simulink model "DARM"  (Simulink 7.5)
settings: Solver=ode45  StartTime=0.0  StopTime=10.0  RelTol=1e-3
values from neighbouring files (symbols this model uses):
  ifoParams = evalin('base', 'ifoParams')    [darmNbParams.m]
libraries: cstblocks x132, NbLibrary x29
(part 1 of 2)
settings Model: Creator=kissel  LastModifiedBy=controls
settings CodeAppCC: CustomSymbolStrType=$N$R$M_T

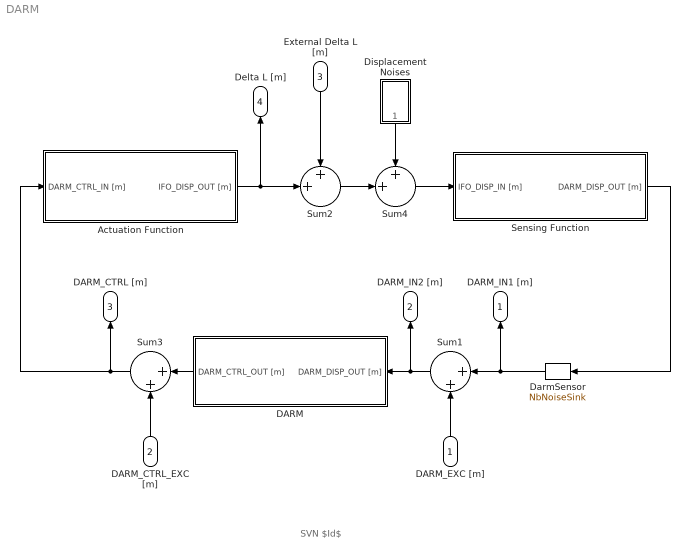
== system DARM ==
  note: SVN $Id$
  DARM_EXC [m] : Inport
  DARM_CTRL_EXC [m] : Inport  Port=2
  External Delta L [m] : Inport  Port=3
  Actuation Function : Subsystem
  DARM : Subsystem
  DarmSensor : NbLibrary/NbNoiseSink  Tag=NbNoiseSink  SystemSampleTime=-1  dof='DARM'
      settings: AttributesFormatString=%<Tag>
  Displacement Noises : Subsystem
  Sensing Function : Subsystem
  Sum1 : Sum  Inputs=|++
  Sum2 : Sum  Inputs=++|
  Sum3 : Sum  Inputs=|++
  Sum4 : Sum  Inputs=++|
  DARM_IN1 [m] : Outport
  DARM_IN2 [m] : Outport  Port=2
  DARM_CTRL [m] : Outport  Port=3
  Delta L [m] : Outport  Port=4
  wires:
  Sum1/1 -> DARM/1(DARM_DISP_OUT [m]), DARM_IN2 [m]/1
  Sensing Function/1(DARM_DISP_OUT [m]) -> DarmSensor/1
  DARM_EXC [m]/1 -> Sum1/2
  Actuation Function/1(IFO_DISP_OUT [m]) -> Sum2/2, Delta L [m]/1
  External Delta L [m]/1 -> Sum2/1
  Sum3/1 -> Actuation Function/1(DARM_CTRL_IN [m]), DARM_CTRL [m]/1
  DARM_CTRL_EXC [m]/1 -> Sum3/2
  DARM/1(DARM_CTRL_OUT [m]) -> Sum3/1
  DarmSensor/1 -> Sum1/1, DARM_IN1 [m]/1
  Sum2/1 -> Sum4/2
  Sum4/1 -> Sensing Function/1(IFO_DISP_IN [m])
  Displacement Noises/1(Out [m]) -> Sum4/1

== system DARM/Actuation Function ==
  DARM_CTRL_IN [m] : Inport
  ETMX : Subsystem
  ETMY : Subsystem
  IFO2OPTIC : Subsystem
  Subtract : Sum  Inputs=+-
  IFO_DISP_OUT [m] : Outport
  wires:
  IFO2OPTIC/1(ETMX_CTRL_OUT [m]) -> ETMX/1(ETMX_CTRL_IN [m])
  IFO2OPTIC/2(ETMY_CTRL_OUT [m]) -> ETMY/1(ETMY_CTRL_IN [m])
  ETMX/1(ETM_Displacement [m]) -> Subtract/1
  ETMY/1(ETM_Displacement [m]) -> Subtract/2
  DARM_CTRL_IN [m]/1 -> IFO2OPTIC/1(DARM_CTRL_IN [m])
  Subtract/1 -> IFO_DISP_OUT [m]/1

== system DARM/DARM ==
  DARM_DISP_OUT [m] : Inport
  FM1 : cstblocks/LTI System  Description=FlexTf: ifoParams.dig.darm(1).frd  SystemSampleTime=-1  sys=ifoParams.dig.darm(1).ss  IC=[]
      settings: AttributesFormatString=%<Description>
  FM10 : cstblocks/LTI System  SystemSampleTime=-1  sys=ifoParams.dig.darm(10).ss  IC=[]
  FM2 : cstblocks/LTI System  Description=FlexTf: ifoParams.dig.darm(2).frd  SystemSampleTime=-1  sys=ifoParams.dig.darm(2).ss  IC=[]
      settings: AttributesFormatString=%<Description>
  FM3 : cstblocks/LTI System  SystemSampleTime=-1  sys=ifoParams.dig.darm(3).ss  IC=[]
  FM4 : cstblocks/LTI System  SystemSampleTime=-1  sys=ifoParams.dig.darm(4).ss  IC=[]
  FM5 : cstblocks/LTI System  SystemSampleTime=-1  sys=ifoParams.dig.darm(5).ss  IC=[]
  FM6 : cstblocks/LTI System  SystemSampleTime=-1  sys=ifoParams.dig.darm(6).ss  IC=[]
  FM7 : cstblocks/LTI System  SystemSampleTime=-1  sys=ifoParams.dig.darm(7).ss  IC=[]
  FM8 : cstblocks/LTI System  SystemSampleTime=-1  sys=ifoParams.dig.darm(8).ss  IC=[]
  FM9 : cstblocks/LTI System  SystemSampleTime=-1  sys=ifoParams.dig.darm(9).ss  IC=[]
  Gain2 : Gain  Gain=ifoParams.dig.darmGain
  DARM_CTRL_OUT [m] : Outport
  wires:
  FM1/1 -> FM2/1
  FM2/1 -> FM3/1
  FM3/1 -> FM4/1
  FM4/1 -> FM5/1
  FM6/1 -> FM7/1
  FM7/1 -> FM8/1
  FM8/1 -> FM9/1
  FM9/1 -> FM10/1
  DARM_DISP_OUT [m]/1 -> FM1/1
  FM10/1 -> Gain2/1
  Gain2/1 -> DARM_CTRL_OUT [m]/1
  FM5/1 -> FM6/1

== system DARM/Displacement Noises ==
  DarmMeters : NbLibrary/NbNoiseCal  Tag=NbNoiseCal  SystemSampleTime=-1  dof='DARM'  unit='displacement [m/rtHz]'
      settings: AttributesFormatString=%<Tag>
  ScatteredLightRing : NbLibrary/NbNoiseSource  Tag=NbNoiseSource  SystemSampleTime=-1  group='Scattered Light Ring'  asd=ifoParams.darmNb.scatteredLightRing
      settings: AttributesFormatString=%<Tag>
  Sum2 : Sum
  Out [m] : Outport
  wires:
  DarmMeters/1 -> Sum2/1
  Sum2/1 -> Out [m]/1
  ScatteredLightRing/1 -> Sum2/2

== system DARM/Sensing Function ==
  IFO_DISP_IN [m] : Inport
  ADC : Subsystem
  DCPD Analog Electronics : Subsystem
  DCPD Signal Conditioning : Subsystem
  IFO2PD : Subsystem
  LaserAm : NbLibrary/NbNoiseSource  Tag=NbNoiseSource  SystemSampleTime=-1  group='Laser Intensity'  asd=ifoParams.darmNb.laserAm
      settings: AttributesFormatString=%<Tag>
  LaserPm : NbLibrary/NbNoiseSource  Tag=NbNoiseSource  SystemSampleTime=-1  group='Laser Frequency'  asd=ifoParams.darmNb.laserPm
      settings: AttributesFormatString=%<Tag>
  Mich : NbLibrary/NbNoiseSource  Tag=NbNoiseSource  SystemSampleTime=-1  group='MICH Coupling'  asd=ifoParams.darmNb.mich
      settings: AttributesFormatString=%<Tag>
  OscAm : NbLibrary/NbNoiseSource  Tag=NbNoiseSource  SystemSampleTime=-1  group='Oscillator Amplitude'  asd=ifoParams.darmNb.oscAm
      settings: AttributesFormatString=%<Tag>
  OscPm : NbLibrary/NbNoiseSource  Tag=NbNoiseSource  SystemSampleTime=-1  group='Oscillator Phase'  asd=ifoParams.darmNb.oscPm
      settings: AttributesFormatString=%<Tag>
  PD2IFO : Subsystem
  Quantum : NbLibrary/NbNoiseSource  Tag=NbNoiseSource  SystemSampleTime=-1  group='Quantum'  asd=ifoParams.darmNb.quantum
      settings: AttributesFormatString=%<Tag>
  Sum2 : Sum  Inputs=+++++++
  ifoResponse : cstblocks/LTI System  Description=FlexTf: ifoParams.sens.ifoResponse.frd  SystemSampleTime=-1  sys=ifoParams.sens.ifoResponse.ss  IC=[]
      settings: AttributesFormatString=%<Description>
  DARM_DISP_OUT [m] : Outport
  wires:
  IFO2PD/1(PD1_OUT [W]) -> DCPD Analog Electronics/1(PD1_IN [W])
  IFO2PD/2(PD2_OUT [W]) -> DCPD Analog Electronics/2(PD2_IN [W])
  IFO_DISP_IN [m]/1 -> ifoResponse/1
  DCPD Signal Conditioning/1(PD1_OUT [m]) -> PD2IFO/1(PD1_IN1 [m])
  DCPD Signal Conditioning/2(PD2_OUT [m]) -> PD2IFO/2(PD2_IN [m])
  PD2IFO/1(DARM_DISP_OUT [m]) -> DARM_DISP_OUT [m]/1
  DCPD Analog Electronics/1(PD1_OUT [V]) -> ADC/1(PD1_IN1 [V])
  DCPD Analog Electronics/2(PD2_OUT [V]) -> ADC/2(PD2_IN [V])
  ADC/1(PD1_OUT [ct]) -> DCPD Signal Conditioning/1(PD1_IN [ct])
  ADC/2(PD2_OUT [ct]) -> DCPD Signal Conditioning/2(PD2_IN [ct])
  ifoResponse/1 -> Sum2/1
  Sum2/1 -> IFO2PD/1(IFO_OUT [W])
  LaserAm/1 -> Sum2/2
  LaserPm/1 -> Sum2/3
  OscAm/1 -> Sum2/4
  OscPm/1 -> Sum2/5
  Quantum/1 -> Sum2/6
  Mich/1 -> Sum2/7

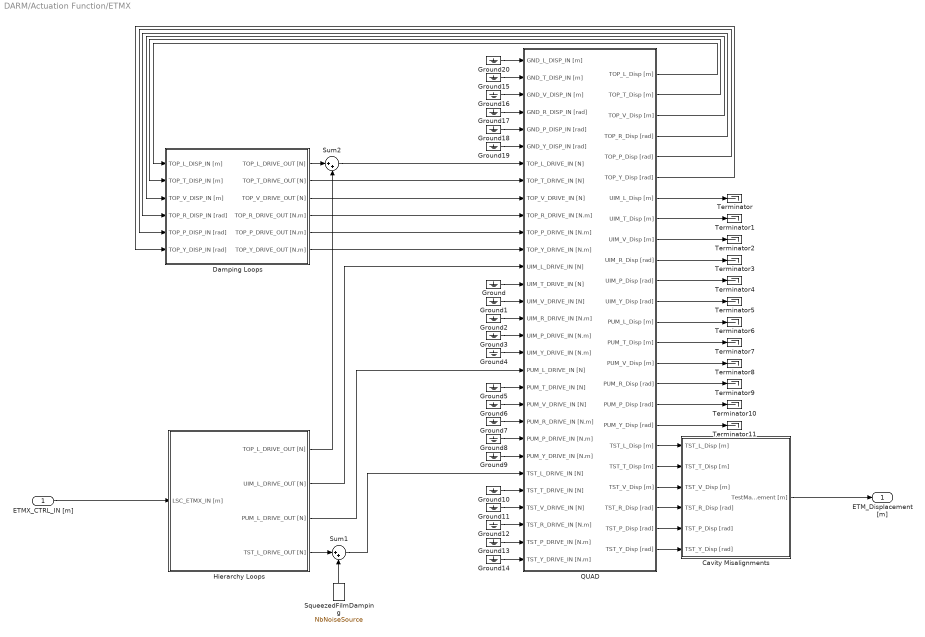
== system DARM/Actuation Function/ETMX ==
  ETMX_CTRL_IN [m] : Inport
  Cavity Misalignments : Subsystem
  Damping Loops : Subsystem
  Ground{,1..20} (21 alike) : Ground
  Hierarchy Loops : Subsystem
  QUAD : Subsystem
  SqueezedFilmDamping : NbLibrary/NbNoiseSource  Tag=NbNoiseSource  SystemSampleTime=-1  group='Squeezed Film Damping'  asd=ifoParams.darmNb.squeezedFilmDamping
      settings: AttributesFormatString=%<Tag>
  Sum1 : Sum  Inputs=|++
  Sum2 : Sum  Inputs=|++
  Terminator{,1..11} (12 alike) : Terminator
  ETM_Displacement [m] : Outport
  wires:
  QUAD/1(TOP_L_Disp [m]) -> Damping Loops/1(TOP_L_DISP_IN [m])
  QUAD/2(TOP_T_Disp [m]) -> Damping Loops/2(TOP_T_DISP_IN [m])
  QUAD/3(TOP_V_Disp [m]) -> Damping Loops/3(TOP_V_DISP_IN [m])
  QUAD/4(TOP_R_Disp [rad]) -> Damping Loops/4(TOP_R_DISP_IN [rad])
  QUAD/5(TOP_P_Disp [rad]) -> Damping Loops/5(TOP_P_DISP_IN [rad])
  QUAD/6(TOP_Y_Disp [rad]) -> Damping Loops/6(TOP_Y_DISP_IN [rad])
  QUAD/7(UIM_L_Disp [m]) -> Terminator/1
  QUAD/8(UIM_T_Disp [m]) -> Terminator1/1
  QUAD/9(UIM_V_Disp [m]) -> Terminator2/1
  QUAD/10(UIM_R_Disp [rad]) -> Terminator3/1
  QUAD/11(UIM_P_Disp [rad]) -> Terminator4/1
  QUAD/12(UIM_Y_Disp [rad]) -> Terminator5/1
  QUAD/13(PUM_L_Disp [m]) -> Terminator6/1
  QUAD/14(PUM_T_Disp [m]) -> Terminator7/1
  QUAD/15(PUM_V_Disp [m]) -> Terminator8/1
  QUAD/16(PUM_R_Disp [rad]) -> Terminator9/1
  QUAD/17(PUM_P_Disp [rad]) -> Terminator10/1
  QUAD/18(PUM_Y_Disp [rad]) -> Terminator11/1
  QUAD/19(TST_L_Disp [m]) -> Cavity Misalignments/1(TST_L_Disp [m])
  QUAD/20(TST_T_Disp [m]) -> Cavity Misalignments/2(TST_T_Disp [m])
  QUAD/21(TST_V_Disp [m]) -> Cavity Misalignments/3(TST_V_Disp [m])
  QUAD/22(TST_R_Disp [rad]) -> Cavity Misalignments/4(TST_R_Disp [rad])
  QUAD/23(TST_P_Disp [rad]) -> Cavity Misalignments/5(TST_P_Disp [rad])
  QUAD/24(TST_Y_Disp [rad]) -> Cavity Misalignments/6(TST_Y_Disp [rad])
  Ground/1 -> QUAD/14(UIM_T_DRIVE_IN [N])
  Ground1/1 -> QUAD/15(UIM_V_DRIVE_IN [N])
  Ground4/1 -> QUAD/18(UIM_Y_DRIVE_IN [N.m])
  Ground3/1 -> QUAD/17(UIM_P_DRIVE_IN [N.m])
  Ground2/1 -> QUAD/16(UIM_R_DRIVE_IN [N.m])
  Ground5/1 -> QUAD/20(PUM_T_DRIVE_IN [N])
  Ground6/1 -> QUAD/21(PUM_V_DRIVE_IN [N])
  Ground7/1 -> QUAD/22(PUM_R_DRIVE_IN [N.m])
  Ground8/1 -> QUAD/23(PUM_P_DRIVE_IN [N.m])
  Ground9/1 -> QUAD/24(PUM_Y_DRIVE_IN [N.m])
  Ground10/1 -> QUAD/26(TST_T_DRIVE_IN [N])
  Ground11/1 -> QUAD/27(TST_V_DRIVE_IN [N])
  Ground12/1 -> QUAD/28(TST_R_DRIVE_IN [N.m])
  Ground13/1 -> QUAD/29(TST_P_DRIVE_IN [N.m])
  Ground14/1 -> QUAD/30(TST_Y_DRIVE_IN [N.m])
  Cavity Misalignments/1(TestMass_L_Displacement [m]) -> ETM_Displacement [m]/1
  Hierarchy Loops/3(PUM_L_DRIVE_OUT [N]) -> QUAD/19(PUM_L_DRIVE_IN [N])
  Hierarchy Loops/2(UIM_L_DRIVE_OUT [N]) -> QUAD/13(UIM_L_DRIVE_IN [N])
  Damping Loops/2(TOP_T_DRIVE_OUT [N]) -> QUAD/8(TOP_T_DRIVE_IN [N])
  Damping Loops/3(TOP_V_DRIVE_OUT [N]) -> QUAD/9(TOP_V_DRIVE_IN [N])
  Damping Loops/4(TOP_R_DRIVE_OUT [N.m]) -> QUAD/10(TOP_R_DRIVE_IN [N.m])
  Damping Loops/5(TOP_P_DRIVE_OUT [N.m]) -> QUAD/11(TOP_P_DRIVE_IN [N.m])
  Damping Loops/6(TOP_Y_DRIVE_OUT [N.m]) -> QUAD/12(TOP_Y_DRIVE_IN [N.m])
  Damping Loops/1(TOP_L_DRIVE_OUT [N]) -> Sum2/1
  Hierarchy Loops/1(TOP_L_DRIVE_OUT [N]) -> Sum2/2
  Sum2/1 -> QUAD/7(TOP_L_DRIVE_IN [N])
  ETMX_CTRL_IN [m]/1 -> Hierarchy Loops/1(LSC_ETMX_IN [m])
  Ground20/1 -> QUAD/1(GND_L_DISP_IN [m])
  Ground15/1 -> QUAD/2(GND_T_DISP_IN [m])
  Ground16/1 -> QUAD/3(GND_V_DISP_IN [m])
  Ground17/1 -> QUAD/4(GND_R_DISP_IN [rad])
  Ground18/1 -> QUAD/5(GND_P_DISP_IN [rad])
  Ground19/1 -> QUAD/6(GND_Y_DISP_IN [rad])
  Sum1/1 -> QUAD/25(TST_L_DRIVE_IN [N])
  Hierarchy Loops/4(TST_L_DRIVE_OUT [N]) -> Sum1/1
  SqueezedFilmDamping/1 -> Sum1/2

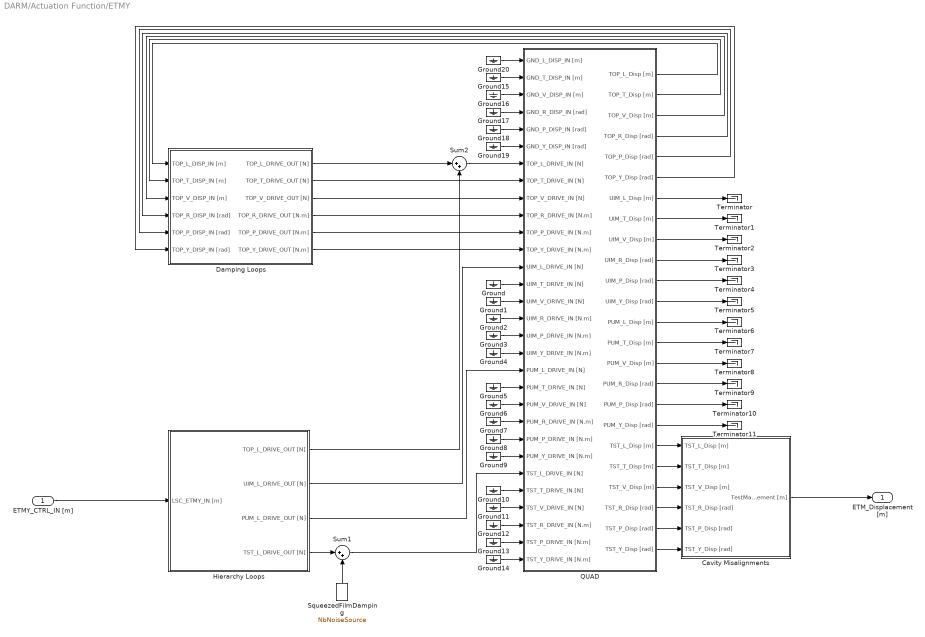
== system DARM/Actuation Function/ETMY ==
  ETMY_CTRL_IN [m] : Inport
  Cavity Misalignments : Subsystem
  Damping Loops : Subsystem
  Ground{,1..20} (21 alike) : Ground
  Hierarchy Loops : Subsystem
  QUAD : Subsystem
  SqueezedFilmDamping : NbLibrary/NbNoiseSource  Tag=NbNoiseSource  SystemSampleTime=-1  group='Squeezed Film Damping'  asd=ifoParams.darmNb.squeezedFilmDamping
      settings: AttributesFormatString=%<Tag>
  Sum1 : Sum  Inputs=|++
  Sum2 : Sum  Inputs=|++
  Terminator{,1..11} (12 alike) : Terminator
  ETM_Displacement [m] : Outport
  wires:
  QUAD/1(TOP_L_Disp [m]) -> Damping Loops/1(TOP_L_DISP_IN [m])
  QUAD/2(TOP_T_Disp [m]) -> Damping Loops/2(TOP_T_DISP_IN [m])
  QUAD/3(TOP_V_Disp [m]) -> Damping Loops/3(TOP_V_DISP_IN [m])
  QUAD/4(TOP_R_Disp [rad]) -> Damping Loops/4(TOP_R_DISP_IN [rad])
  QUAD/5(TOP_P_Disp [rad]) -> Damping Loops/5(TOP_P_DISP_IN [rad])
  QUAD/6(TOP_Y_Disp [rad]) -> Damping Loops/6(TOP_Y_DISP_IN [rad])
  QUAD/7(UIM_L_Disp [m]) -> Terminator/1
  QUAD/8(UIM_T_Disp [m]) -> Terminator1/1
  QUAD/9(UIM_V_Disp [m]) -> Terminator2/1
  QUAD/10(UIM_R_Disp [rad]) -> Terminator3/1
  QUAD/11(UIM_P_Disp [rad]) -> Terminator4/1
  QUAD/12(UIM_Y_Disp [rad]) -> Terminator5/1
  QUAD/13(PUM_L_Disp [m]) -> Terminator6/1
  QUAD/14(PUM_T_Disp [m]) -> Terminator7/1
  QUAD/15(PUM_V_Disp [m]) -> Terminator8/1
  QUAD/16(PUM_R_Disp [rad]) -> Terminator9/1
  QUAD/17(PUM_P_Disp [rad]) -> Terminator10/1
  QUAD/18(PUM_Y_Disp [rad]) -> Terminator11/1
  QUAD/19(TST_L_Disp [m]) -> Cavity Misalignments/1(TST_L_Disp [m])
  QUAD/20(TST_T_Disp [m]) -> Cavity Misalignments/2(TST_T_Disp [m])
  QUAD/21(TST_V_Disp [m]) -> Cavity Misalignments/3(TST_V_Disp [m])
  QUAD/22(TST_R_Disp [rad]) -> Cavity Misalignments/4(TST_R_Disp [rad])
  QUAD/23(TST_P_Disp [rad]) -> Cavity Misalignments/5(TST_P_Disp [rad])
  QUAD/24(TST_Y_Disp [rad]) -> Cavity Misalignments/6(TST_Y_Disp [rad])
  Ground/1 -> QUAD/14(UIM_T_DRIVE_IN [N])
  Ground1/1 -> QUAD/15(UIM_V_DRIVE_IN [N])
  Ground4/1 -> QUAD/18(UIM_Y_DRIVE_IN [N.m])
  Ground3/1 -> QUAD/17(UIM_P_DRIVE_IN [N.m])
  Ground2/1 -> QUAD/16(UIM_R_DRIVE_IN [N.m])
  Ground5/1 -> QUAD/20(PUM_T_DRIVE_IN [N])
  Ground6/1 -> QUAD/21(PUM_V_DRIVE_IN [N])
  Ground7/1 -> QUAD/22(PUM_R_DRIVE_IN [N.m])
  Ground8/1 -> QUAD/23(PUM_P_DRIVE_IN [N.m])
  Ground9/1 -> QUAD/24(PUM_Y_DRIVE_IN [N.m])
  Ground10/1 -> QUAD/26(TST_T_DRIVE_IN [N])
  Ground11/1 -> QUAD/27(TST_V_DRIVE_IN [N])
  Ground12/1 -> QUAD/28(TST_R_DRIVE_IN [N.m])
  Ground13/1 -> QUAD/29(TST_P_DRIVE_IN [N.m])
  Ground14/1 -> QUAD/30(TST_Y_DRIVE_IN [N.m])
  Cavity Misalignments/1(TestMass_L_Displacement [m]) -> ETM_Displacement [m]/1
  Hierarchy Loops/3(PUM_L_DRIVE_OUT [N]) -> QUAD/19(PUM_L_DRIVE_IN [N])
  Hierarchy Loops/2(UIM_L_DRIVE_OUT [N]) -> QUAD/13(UIM_L_DRIVE_IN [N])
  Damping Loops/2(TOP_T_DRIVE_OUT [N]) -> QUAD/8(TOP_T_DRIVE_IN [N])
  Damping Loops/3(TOP_V_DRIVE_OUT [N]) -> QUAD/9(TOP_V_DRIVE_IN [N])
  Damping Loops/4(TOP_R_DRIVE_OUT [N.m]) -> QUAD/10(TOP_R_DRIVE_IN [N.m])
  Damping Loops/5(TOP_P_DRIVE_OUT [N.m]) -> QUAD/11(TOP_P_DRIVE_IN [N.m])
  Damping Loops/6(TOP_Y_DRIVE_OUT [N.m]) -> QUAD/12(TOP_Y_DRIVE_IN [N.m])
  Damping Loops/1(TOP_L_DRIVE_OUT [N]) -> Sum2/1
  Hierarchy Loops/1(TOP_L_DRIVE_OUT [N]) -> Sum2/2
  Sum2/1 -> QUAD/7(TOP_L_DRIVE_IN [N])
  ETMY_CTRL_IN [m]/1 -> Hierarchy Loops/1(LSC_ETMY_IN [m])
  Ground20/1 -> QUAD/1(GND_L_DISP_IN [m])
  Ground15/1 -> QUAD/2(GND_T_DISP_IN [m])
  Ground16/1 -> QUAD/3(GND_V_DISP_IN [m])
  Ground17/1 -> QUAD/4(GND_R_DISP_IN [rad])
  Ground18/1 -> QUAD/5(GND_P_DISP_IN [rad])
  Ground19/1 -> QUAD/6(GND_Y_DISP_IN [rad])
  Hierarchy Loops/4(TST_L_DRIVE_OUT [N]) -> Sum1/1
  SqueezedFilmDamping/1 -> Sum1/2
  Sum1/1 -> QUAD/25(TST_L_DRIVE_IN [N])

== system DARM/Actuation Function/IFO2OPTIC ==
  DARM_CTRL_IN [m] : Inport
  Gain3 : Gain  Gain=ifoParams.act.darm2etmx
  Gain4 : Gain  Gain=ifoParams.act.darm2etmy
  ETMX_CTRL_OUT [m] : Outport
  ETMY_CTRL_OUT [m] : Outport  Port=2
  wires:
  DARM_CTRL_IN [m]/1 -> Gain3/1, Gain4/1
  Gain3/1 -> ETMX_CTRL_OUT [m]/1
  Gain4/1 -> ETMY_CTRL_OUT [m]/1

== system DARM/Sensing Function/ADC ==
  note: ifoParams.sens.adcGain
      | [ct/V]
  PD1_IN1 [V] : Inport
  PD2_IN [V] : Inport  Port=2
  AdcPd1 : NbLibrary/NbNoiseSource  Tag=NbNoiseSource  SystemSampleTime=-1  group='ADC'  asd=ifoParams.darmNb.adc
      settings: AttributesFormatString=%<Tag>
  AdcPd2 : NbLibrary/NbNoiseSource  Tag=NbNoiseSource  SystemSampleTime=-1  group='ADC'  asd=ifoParams.darmNb.adc
      settings: AttributesFormatString=%<Tag>
  Gain1 : Gain  Gain=ifoParams.sens.adcGain
  Gain3 : Gain  Gain=ifoParams.sens.adcGain
  Sum2 : Sum  Inputs=++|
  Sum3 : Sum  Inputs=|++
  PD1_OUT [ct] : Outport
  PD2_OUT [ct] : Outport  Port=2
  wires:
  AdcPd1/1 -> Sum2/1
  PD1_IN1 [V]/1 -> Sum2/2
  Sum2/1 -> Gain3/1
  Gain3/1 -> PD1_OUT [ct]/1
  AdcPd2/1 -> Sum3/2
  PD2_IN [V]/1 -> Sum3/1
  Sum3/1 -> Gain1/1
  Gain1/1 -> PD2_OUT [ct]/1

== system DARM/Sensing Function/DCPD Analog Electronics ==
  PD1_IN [W] : Inport
  PD2_IN [W] : Inport  Port=2
  Anti-Aliasing Chassis : Subsystem
  Aspd1Dark : NbLibrary/NbNoiseSource  Tag=NbNoiseSource  SystemSampleTime=-1  group='ASPD Dark'  asd=ifoParams.darmNb.aspdDark
      settings: AttributesFormatString=%<Tag>
  Aspd2Dark : NbLibrary/NbNoiseSource  Tag=NbNoiseSource  SystemSampleTime=-1  group='ASPD Dark'  asd=ifoParams.darmNb.aspdDark
      settings: AttributesFormatString=%<Tag>
  PD Quantum Efficiency : Subsystem
  Preamps : Subsystem
  Sum1 : Sum  Inputs=|++
  Sum2 : Sum  Inputs=++|
  Whitening Chassis : Subsystem
  PD1_OUT [V] : Outport
  PD2_OUT [V] : Outport  Port=2
  wires:
  Preamps/1(PD1_OUT [V]) -> Whitening Chassis/1(PD1_IN1 [V])
  Preamps/2(PD2_OUT [V]) -> Whitening Chassis/2(PD2_IN [V])
  Whitening Chassis/1(PD1_OUT [V]) -> Anti-Aliasing Chassis/1(PD1_IN1 [V])
  Whitening Chassis/2(PD2_OUT [V]) -> Anti-Aliasing Chassis/2(PD2_IN [V])
  Anti-Aliasing Chassis/1(PD1_OUT [V]) -> PD1_OUT [V]/1
  PD1_IN [W]/1 -> PD Quantum Efficiency/1(PD1_IN1 [W])
  Anti-Aliasing Chassis/2(PD2_OUT [V]) -> PD2_OUT [V]/1
  PD2_IN [W]/1 -> PD Quantum Efficiency/2(PD2_IN [W])
  PD Quantum Efficiency/1(PD1_OUT [A]) -> Sum2/2
  PD Quantum Efficiency/2(PD2_OUT [A]) -> Sum1/1
  Sum2/1 -> Preamps/1(PD1_IN1 [A])
  Sum1/1 -> Preamps/2(PD2_IN [A])
  Aspd1Dark/1 -> Sum2/1
  Aspd2Dark/1 -> Sum1/2

== system DARM/Sensing Function/DCPD Signal Conditioning ==
  PD1_IN [ct] : Inport
  PD2_IN [ct] : Inport  Port=2
  64k to 16k Downsampling Filter : Subsystem
  ISCINF : Subsystem
  PD1_OUT [m] : Outport
  PD2_OUT [m] : Outport  Port=2
  wires:
  64k to 16k Downsampling Filter/1(PD1_OUT [ct]) -> ISCINF/1(PD1_IN [ct])
  64k to 16k Downsampling Filter/2(PD2_OUT [ct]) -> ISCINF/2(PD2_IN [ct])
  PD1_IN [ct]/1 -> 64k to 16k Downsampling Filter/1(PDq_IN [ct])
  ISCINF/1(PD1_OUT [m]) -> PD1_OUT [m]/1
  PD2_IN [ct]/1 -> 64k to 16k Downsampling Filter/2(PD2_IN [ct])
  ISCINF/2(PD2_OUT [m]) -> PD2_OUT [m]/1

== system DARM/Sensing Function/IFO2PD ==
  IFO_OUT [W] : Inport
  Gain2 : Gain  Gain=ifoParams.sens.ifo2pd1
  Gain4 : Gain  Gain=ifoParams.sens.ifo2pd2
  PD1_OUT [W] : Outport
  PD2_OUT [W] : Outport  Port=2
  wires:
  IFO_OUT [W]/1 -> Gain2/1, Gain4/1
  Gain2/1 -> PD1_OUT [W]/1
  Gain4/1 -> PD2_OUT [W]/1

== system DARM/Sensing Function/PD2IFO ==
  PD1_IN1 [m] : Inport
  PD2_IN [m] : Inport  Port=2
  Sum2 : Sum
  DARM_DISP_OUT [m] : Outport
  wires:
  PD1_IN1 [m]/1 -> Sum2/1
  Sum2/1 -> DARM_DISP_OUT [m]/1
  PD2_IN [m]/1 -> Sum2/2

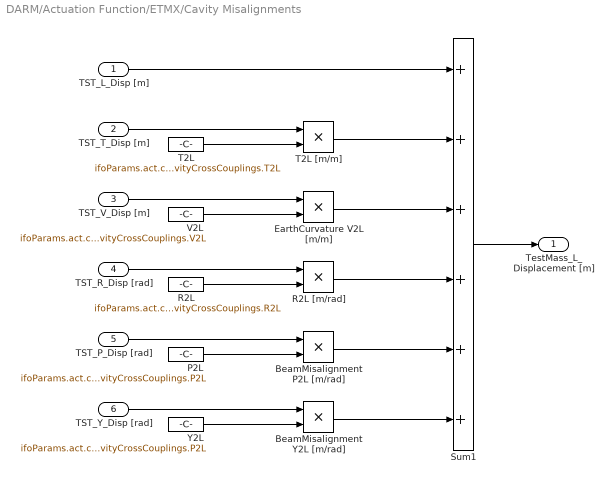
== system DARM/Actuation Function/ETMX/Cavity Misalignments ==
  TST_L_Disp [m] : Inport
  TST_T_Disp [m] : Inport  Port=2
  TST_V_Disp [m] : Inport  Port=3
  TST_R_Disp [rad] : Inport  Port=4
  TST_P_Disp [rad] : Inport  Port=5
  TST_Y_Disp [rad] : Inport  Port=6
  BeamMisalignment P2L [m/rad] : Product  RndMeth=Zero
  BeamMisalignment Y2L [m/rad] : Product  RndMeth=Zero
  EarthCurvature V2L [m/m] : Product  RndMeth=Zero
  P2L : Constant  Value=ifoParams.act.cavityCrossCouplings.P2L
  R2L : Constant  Value=ifoParams.act.cavityCrossCouplings.R2L
  R2L [m/rad] : Product  RndMeth=Zero
  Sum1 : Sum  Inputs=++++++
  T2L : Constant  Value=ifoParams.act.cavityCrossCouplings.T2L
  T2L [m/m] : Product  RndMeth=Zero
  V2L : Constant  Value=ifoParams.act.cavityCrossCouplings.V2L
  Y2L : Constant  Value=ifoParams.act.cavityCrossCouplings.P2L
  TestMass_L_Displacement [m] : Outport
  wires:
  V2L/1 -> EarthCurvature V2L [m/m]/2
  P2L/1 -> BeamMisalignment P2L [m/rad]/2
  Y2L/1 -> BeamMisalignment Y2L [m/rad]/2
  TST_V_Disp [m]/1 -> EarthCurvature V2L [m/m]/1
  TST_P_Disp [rad]/1 -> BeamMisalignment P2L [m/rad]/1
  TST_Y_Disp [rad]/1 -> BeamMisalignment Y2L [m/rad]/1
  R2L/1 -> R2L [m/rad]/2
  T2L/1 -> T2L [m/m]/2
  TST_R_Disp [rad]/1 -> R2L [m/rad]/1
  TST_T_Disp [m]/1 -> T2L [m/m]/1
  Sum1/1 -> TestMass_L_Displacement [m]/1
  TST_L_Disp [m]/1 -> Sum1/1
  T2L [m/m]/1 -> Sum1/2
  EarthCurvature V2L [m/m]/1 -> Sum1/3
  R2L [m/rad]/1 -> Sum1/4
  BeamMisalignment P2L [m/rad]/1 -> Sum1/5
  BeamMisalignment Y2L [m/rad]/1 -> Sum1/6

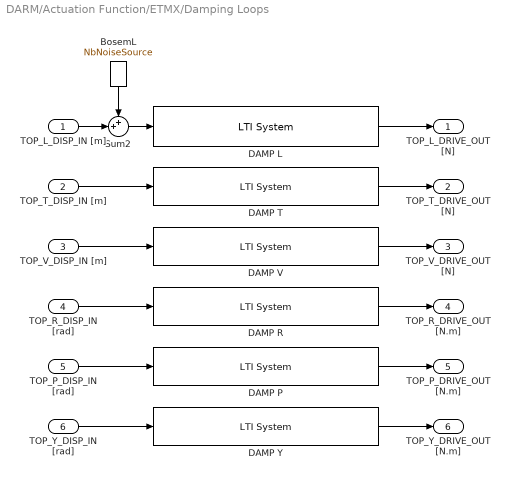
== system DARM/Actuation Function/ETMX/Damping Loops ==
  TOP_L_DISP_IN [m] : Inport
  TOP_T_DISP_IN [m] : Inport  Port=2
  TOP_V_DISP_IN [m] : Inport  Port=3
  TOP_R_DISP_IN [rad] : Inport  Port=4
  TOP_P_DISP_IN [rad] : Inport  Port=5
  TOP_Y_DISP_IN [rad] : Inport  Port=6
  BosemL : NbLibrary/NbNoiseSource  Tag=NbNoiseSource  SystemSampleTime=-1  group='BOSEM L'  asd=ifoParams.darmNb.bosem
      settings: AttributesFormatString=%<Tag>
  DAMP L : cstblocks/LTI System  SystemSampleTime=-1  sys=ifoParams.act.damp(1).ss  IC=[]
  DAMP P : cstblocks/LTI System  SystemSampleTime=-1  sys=ifoParams.act.damp(5).ss  IC=[]
  DAMP R : cstblocks/LTI System  SystemSampleTime=-1  sys=ifoParams.act.damp(4).ss  IC=[]
  DAMP T : cstblocks/LTI System  SystemSampleTime=-1  sys=ifoParams.act.damp(2).ss  IC=[]
  DAMP V : cstblocks/LTI System  SystemSampleTime=-1  sys=ifoParams.act.damp(3).ss  IC=[]
  DAMP Y : cstblocks/LTI System  SystemSampleTime=-1  sys=ifoParams.act.damp(6).ss  IC=[]
  Sum2 : Sum  Inputs=++|
  TOP_L_DRIVE_OUT [N] : Outport
  TOP_T_DRIVE_OUT [N] : Outport  Port=2
  TOP_V_DRIVE_OUT [N] : Outport  Port=3
  TOP_R_DRIVE_OUT [N.m] : Outport  Port=4
  TOP_P_DRIVE_OUT [N.m] : Outport  Port=5
  TOP_Y_DRIVE_OUT [N.m] : Outport  Port=6
  wires:
  DAMP L/1 -> TOP_L_DRIVE_OUT [N]/1
  DAMP T/1 -> TOP_T_DRIVE_OUT [N]/1
  DAMP V/1 -> TOP_V_DRIVE_OUT [N]/1
  DAMP R/1 -> TOP_R_DRIVE_OUT [N.m]/1
  DAMP P/1 -> TOP_P_DRIVE_OUT [N.m]/1
  DAMP Y/1 -> TOP_Y_DRIVE_OUT [N.m]/1
  TOP_T_DISP_IN [m]/1 -> DAMP T/1
  TOP_V_DISP_IN [m]/1 -> DAMP V/1
  TOP_R_DISP_IN [rad]/1 -> DAMP R/1
  TOP_P_DISP_IN [rad]/1 -> DAMP P/1
  TOP_Y_DISP_IN [rad]/1 -> DAMP Y/1
  TOP_L_DISP_IN [m]/1 -> Sum2/2
  Sum2/1 -> DAMP L/1
  BosemL/1 -> Sum2/1

== system DARM/Actuation Function/ETMX/Hierarchy Loops ==
  LSC_ETMX_IN [m] : Inport
  Actuator-to-Euler Transform : Subsystem
  Anti-Aliasing Chassis : Subsystem
  COILOUTF : Subsystem
  DAC : Subsystem
  Driver Electronics : Subsystem
  Driver Force Coefficient : Subsystem
  EUL2OSEM : Subsystem
  L1 LOCK : Subsystem
  L2 LOCK : Subsystem
  L3 LOCK : Subsystem
  LSC_ETMX : Subsystem
  M0 LOCK : Subsystem
  esdBias_ct : Constant  Value=ifoParams.act.esdBias_ct
  TOP_L_DRIVE_OUT [N] : Outport
  UIM_L_DRIVE_OUT [N] : Outport  Port=2
  PUM_L_DRIVE_OUT [N] : Outport  Port=3
  TST_L_DRIVE_OUT [N] : Outport  Port=4
  wires:
  Driver Force Coefficient/1(TOP_Out [N]) -> Actuator-to-Euler Transform/1(TOP_OSEM_IN [N])
  Driver Force Coefficient/2(UIM_Out [N]) -> Actuator-to-Euler Transform/2(UIM_OSEM_IN [N])
  Driver Force Coefficient/3(PUM_Out [N]) -> Actuator-to-Euler Transform/3(PUM_OSEM_IN [N])
  Driver Force Coefficient/4(TST_Out [N]) -> Actuator-to-Euler Transform/4(TST_OSEM_IN [N])
  DAC/1(TOP Out [V]) -> Anti-Aliasing Chassis/1(TOP In [V[)
  DAC/2(UIM Out [V]) -> Anti-Aliasing Chassis/2(UIM In [V])
  DAC/3(PUM Out[V]) -> Anti-Aliasing Chassis/3(PUM In [V])
  DAC/4(ESD Ctrl Out V]) -> Anti-Aliasing Chassis/4(ESD Ctrl In [V])
  DAC/5(ESD Bias Out [V]) -> Anti-Aliasing Chassis/5(ESD Bias In [V])
  COILOUTF/1(M0_OUT [ct]) -> DAC/1(M0 In [cts])
  COILOUTF/2(L1_OUT [ct]) -> DAC/2(L1 In [cts])
  COILOUTF/3(L2_OUT [ct]) -> DAC/3(L2 In [cts])
  COILOUTF/4(L3_CTRL_OUT [ct]) -> DAC/4(L3 Ctrl In [cts])
  COILOUTF/5(L3_BIAS_OUT [ct]) -> DAC/5(L3 Bias In [cts])
  M0 LOCK/1(M0_OUT [ct]) -> EUL2OSEM/1(M0_L_IN [ct])
  EUL2OSEM/1(M0_OSEM_OUT [ct]) -> COILOUTF/1(M0_IN [ct])
  EUL2OSEM/2(L1_OSEM_OUT [ct]) -> COILOUTF/2(L1_IN [ct])
  EUL2OSEM/3(L2_OSEM_OUT [ct]) -> COILOUTF/3(L2_IN [ct])
  EUL2OSEM/4(L3_OSEM_OUT [ct]) -> COILOUTF/4(L3_CTRL_IN [ct])
  esdBias_ct/1 -> COILOUTF/5(L3_BIAS_IN [ct])
  LSC_ETMX_IN [m]/1 -> LSC_ETMX/1(LSC_ETMX_IN)
  Actuator-to-Euler Transform/1(TOP_L_OUT [N]) -> TOP_L_DRIVE_OUT [N]/1
  Actuator-to-Euler Transform/2(UIM_L_OUT [N]) -> UIM_L_DRIVE_OUT [N]/1
  Actuator-to-Euler Transform/3(PUM_L_OUT [N]) -> PUM_L_DRIVE_OUT [N]/1
  Actuator-to-Euler Transform/4(TST_L_OUT [N]) -> TST_L_DRIVE_OUT [N]/1
  Anti-Aliasing Chassis/1(TOP Out [V]) -> Driver Electronics/1(TOP In [V])
  Anti-Aliasing Chassis/2(UIM Out [V]) -> Driver Electronics/2(UIM In [V])
  Anti-Aliasing Chassis/3(PUM Out[V]) -> Driver Electronics/3(PUM In [V])
  Anti-Aliasing Chassis/4(ESD Ctrl Out V]) -> Driver Electronics/4(ESD Ctrl In [V])
  Anti-Aliasing Chassis/5(ESD Bias Out [V]) -> Driver Electronics/5(ESD Bias In [V])
  Driver Electronics/1(TOP Out [A]) -> Driver Force Coefficient/1(In1[A])
  Driver Electronics/2(UIM Out [A]) -> Driver Force Coefficient/2(In2[A])
  Driver Electronics/3(PUM Out [A]) -> Driver Force Coefficient/3(In3[A])
  Driver Electronics/4(ESD Ctrl Out[V]) -> Driver Force Coefficient/4(Vsig[V])
  Driver Electronics/5(ESD Bias Out[V]) -> Driver Force Coefficient/5(Vbias[V])
  L1 LOCK/1(L1_OUT [ct]) -> EUL2OSEM/2(L1_L_IN [ct])
  L2 LOCK/1(L2_OUT [ct]) -> EUL2OSEM/3(L2_L_IN [ct])
  L3 LOCK/1(L3_OUT [ct]) -> EUL2OSEM/4(L3_L_IN [ct])
  LSC_ETMX/1("LSC_ETMX_OUT ") -> M0 LOCK/1(LSC_IN [m]), L1 LOCK/1(LSC_IN [m]), L2 LOCK/1(LSC_IN [m]), L3 LOCK/1(LSC_IN [m])

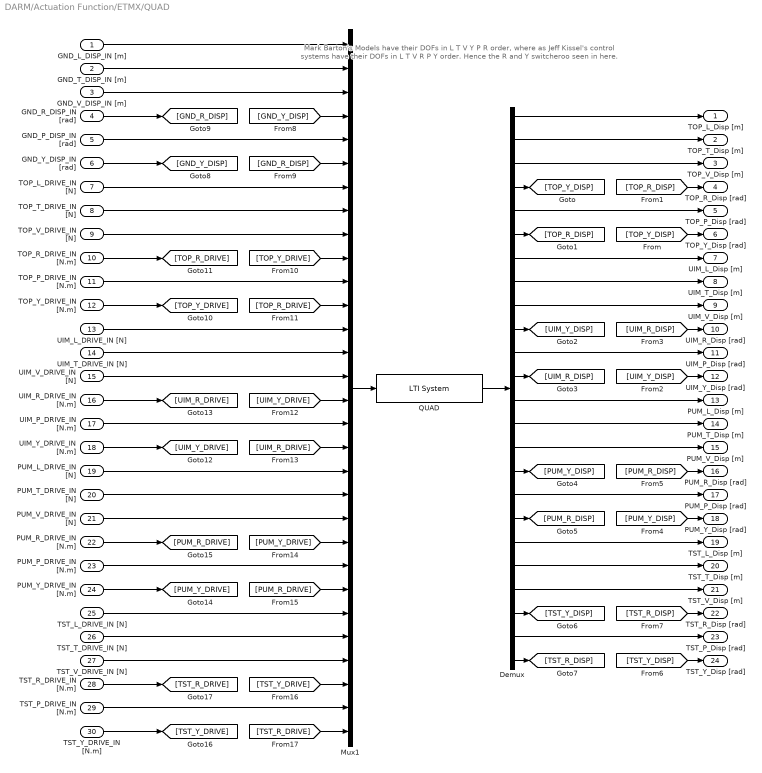
== system DARM/Actuation Function/ETMX/QUAD ==
  note: Mark Barton's Models have their DOFs in
      | L T V Y P R order, where as Jeff Kissel's control
      | systems have their DOFs in  L T V R P Y order.
      | Hence the R and Y switcheroo seen in here.
  GND_L_DISP_IN [m] : Inport
  GND_T_DISP_IN [m] : Inport  Port=2
  GND_V_DISP_IN [m] : Inport  Port=3
  GND_R_DISP_IN [rad] : Inport  Port=4
  GND_P_DISP_IN [rad] : Inport  Port=5
  GND_Y_DISP_IN [rad] : Inport  Port=6
  TOP_L_DRIVE_IN [N] : Inport  Port=7
  TOP_T_DRIVE_IN [N] : Inport  Port=8
  TOP_V_DRIVE_IN [N] : Inport  Port=9
  TOP_R_DRIVE_IN [N.m] : Inport  Port=10
  TOP_P_DRIVE_IN [N.m] : Inport  Port=11
  TOP_Y_DRIVE_IN [N.m] : Inport  Port=12
  UIM_L_DRIVE_IN [N] : Inport  Port=13
  UIM_T_DRIVE_IN [N] : Inport  Port=14
  UIM_V_DRIVE_IN [N] : Inport  Port=15
  UIM_R_DRIVE_IN [N.m] : Inport  Port=16
  UIM_P_DRIVE_IN [N.m] : Inport  Port=17
  UIM_Y_DRIVE_IN [N.m] : Inport  Port=18
  PUM_L_DRIVE_IN [N] : Inport  Port=19
  PUM_T_DRIVE_IN [N] : Inport  Port=20
  PUM_V_DRIVE_IN [N] : Inport  Port=21
  PUM_R_DRIVE_IN [N.m] : Inport  Port=22
  PUM_P_DRIVE_IN [N.m] : Inport  Port=23
  PUM_Y_DRIVE_IN [N.m] : Inport  Port=24
  TST_L_DRIVE_IN [N] : Inport  Port=25
  TST_T_DRIVE_IN [N] : Inport  Port=26
  TST_V_DRIVE_IN [N] : Inport  Port=27
  TST_R_DRIVE_IN [N.m] : Inport  Port=28
  TST_P_DRIVE_IN [N.m] : Inport  Port=29
  TST_Y_DRIVE_IN [N.m] : Inport  Port=30
  Demux : Demux  Outputs=24
  Mux1 : Mux  Inputs=30
  QUAD : cstblocks/LTI System  Description=FlexTf: ifoParams.act.quadModel.frd  SystemSampleTime=-1  sys=ifoParams.act.quadModel.ss  IC=[]
      settings: AttributesFormatString=%<Description>
  TOP_L_Disp [m] : Outport
  TOP_T_Disp [m] : Outport  Port=2
  TOP_V_Disp [m] : Outport  Port=3
  TOP_R_Disp [rad] : Outport  Port=4
  TOP_P_Disp [rad] : Outport  Port=5
  TOP_Y_Disp [rad] : Outport  Port=6
  UIM_L_Disp [m] : Outport  Port=7
  UIM_T_Disp [m] : Outport  Port=8
  UIM_V_Disp [m] : Outport  Port=9
  UIM_R_Disp [rad] : Outport  Port=10
  UIM_P_Disp [rad] : Outport  Port=11
  UIM_Y_Disp [rad] : Outport  Port=12
  PUM_L_Disp [m] : Outport  Port=13
  PUM_T_Disp [m] : Outport  Port=14
  PUM_V_Disp [m] : Outport  Port=15
  PUM_R_Disp [rad] : Outport  Port=16
  PUM_P_Disp [rad] : Outport  Port=17
  PUM_Y_Disp [rad] : Outport  Port=18
  TST_L_Disp [m] : Outport  Port=19
  TST_T_Disp [m] : Outport  Port=20
  TST_V_Disp [m] : Outport  Port=21
  TST_R_Disp [rad] : Outport  Port=22
  TST_P_Disp [rad] : Outport  Port=23
  TST_Y_Disp [rad] : Outport  Port=24
  wires:
  QUAD/1 -> Demux/1
  Mux1/1 -> QUAD/1
  GND_L_DISP_IN [m]/1 -> Mux1/1
  GND_T_DISP_IN [m]/1 -> Mux1/2
  GND_V_DISP_IN [m]/1 -> Mux1/3
  Demux/1 -> TOP_L_Disp [m]/1
  Demux/2 -> TOP_T_Disp [m]/1
  Demux/3 -> TOP_V_Disp [m]/1
  TOP_L_DRIVE_IN [N]/1 -> Mux1/7
  TOP_T_DRIVE_IN [N]/1 -> Mux1/8
  TOP_V_DRIVE_IN [N]/1 -> Mux1/9
  Demux/7 -> UIM_L_Disp [m]/1
  Demux/8 -> UIM_T_Disp [m]/1
  Demux/9 -> UIM_V_Disp [m]/1
  UIM_T_DRIVE_IN [N]/1 -> Mux1/14
  UIM_V_DRIVE_IN [N]/1 -> Mux1/15
  Demux/13 -> PUM_L_Disp [m]/1
  Demux/14 -> PUM_T_Disp [m]/1
  Demux/15 -> PUM_V_Disp [m]/1
  PUM_L_DRIVE_IN [N]/1 -> Mux1/19
  PUM_T_DRIVE_IN [N]/1 -> Mux1/20
  PUM_V_DRIVE_IN [N]/1 -> Mux1/21
  Demux/19 -> TST_L_Disp [m]/1
  Demux/20 -> TST_T_Disp [m]/1
  Demux/21 -> TST_V_Disp [m]/1
  TST_L_DRIVE_IN [N]/1 -> Mux1/25
  TST_T_DRIVE_IN [N]/1 -> Mux1/26
  TST_V_DRIVE_IN [N]/1 -> Mux1/27
  Demux/4 -> [TOP_Y_DISP]
  [TOP_Y_DISP] -> TOP_Y_Disp [rad]/1
  Demux/6 -> [TOP_R_DISP]
  [TOP_R_DISP] -> TOP_R_Disp [rad]/1
  Demux/5 -> TOP_P_Disp [rad]/1
  Demux/10 -> [UIM_Y_DISP]
  Demux/11 -> UIM_P_Disp [rad]/1
  [UIM_R_DISP] -> UIM_R_Disp [rad]/1
  Demux/12 -> [UIM_R_DISP]
  [UIM_Y_DISP] -> UIM_Y_Disp [rad]/1
  Demux/16 -> [PUM_Y_DISP]
  [PUM_R_DISP] -> PUM_R_Disp [rad]/1
  Demux/17 -> PUM_P_Disp [rad]/1
  Demux/18 -> [PUM_R_DISP]
  [PUM_Y_DISP] -> PUM_Y_Disp [rad]/1
  [TST_R_DISP] -> TST_R_Disp [rad]/1
  Demux/22 -> [TST_Y_DISP]
  Demux/23 -> TST_P_Disp [rad]/1
  Demux/24 -> [TST_R_DISP]
  [TST_Y_DISP] -> TST_Y_Disp [rad]/1
  UIM_L_DRIVE_IN [N]/1 -> Mux1/13
  GND_R_DISP_IN [rad]/1 -> [GND_R_DISP]
  [GND_Y_DISP] -> Mux1/4
  GND_P_DISP_IN [rad]/1 -> Mux1/5
  GND_Y_DISP_IN [rad]/1 -> [GND_Y_DISP]
  [GND_R_DISP] -> Mux1/6
  TOP_R_DRIVE_IN [N.m]/1 -> [TOP_R_DRIVE]
  TOP_P_DRIVE_IN [N.m]/1 -> Mux1/11
  TOP_Y_DRIVE_IN [N.m]/1 -> [TOP_Y_DRIVE]
  [TOP_Y_DRIVE] -> Mux1/10
  [TOP_R_DRIVE] -> Mux1/12
  UIM_R_DRIVE_IN [N.m]/1 -> [UIM_R_DRIVE]
  UIM_Y_DRIVE_IN [N.m]/1 -> [UIM_Y_DRIVE]
  PUM_R_DRIVE_IN [N.m]/1 -> [PUM_R_DRIVE]
  PUM_Y_DRIVE_IN [N.m]/1 -> [PUM_Y_DRIVE]
  TST_R_DRIVE_IN [N.m]/1 -> [TST_R_DRIVE]
  TST_Y_DRIVE_IN [N.m]/1 -> [TST_Y_DRIVE]
  [UIM_Y_DRIVE] -> Mux1/16
  UIM_P_DRIVE_IN [N.m]/1 -> Mux1/17
  [UIM_R_DRIVE] -> Mux1/18
  [PUM_Y_DRIVE] -> Mux1/22
  PUM_P_DRIVE_IN [N.m]/1 -> Mux1/23
  [PUM_R_DRIVE] -> Mux1/24
  [TST_Y_DRIVE] -> Mux1/28
  TST_P_DRIVE_IN [N.m]/1 -> Mux1/29
  [TST_R_DRIVE] -> Mux1/30

== system DARM/Actuation Function/ETMY/Cavity Misalignments ==
  TST_L_Disp [m] : Inport
  TST_T_Disp [m] : Inport  Port=2
  TST_V_Disp [m] : Inport  Port=3
  TST_R_Disp [rad] : Inport  Port=4
  TST_P_Disp [rad] : Inport  Port=5
  TST_Y_Disp [rad] : Inport  Port=6
  BeamMisalignment P2L [m/rad] : Product  RndMeth=Zero
  BeamMisalignment Y2L [m/rad] : Product  RndMeth=Zero
  EarthCurvature V2L [m/m] : Product  RndMeth=Zero
  P2L : Constant  Value=ifoParams.act.cavityCrossCouplings.P2L
  R2L : Constant  Value=ifoParams.act.cavityCrossCouplings.R2L
  R2L [m/rad] : Product  RndMeth=Zero
  Sum1 : Sum  Inputs=++++++
  T2L : Constant  Value=ifoParams.act.cavityCrossCouplings.T2L
  T2L [m/m] : Product  RndMeth=Zero
  V2L : Constant  Value=ifoParams.act.cavityCrossCouplings.V2L
  Y2L : Constant  Value=ifoParams.act.cavityCrossCouplings.P2L
  TestMass_L_Displacement [m] : Outport
  wires:
  V2L/1 -> EarthCurvature V2L [m/m]/2
  P2L/1 -> BeamMisalignment P2L [m/rad]/2
  Y2L/1 -> BeamMisalignment Y2L [m/rad]/2
  TST_V_Disp [m]/1 -> EarthCurvature V2L [m/m]/1
  TST_P_Disp [rad]/1 -> BeamMisalignment P2L [m/rad]/1
  TST_Y_Disp [rad]/1 -> BeamMisalignment Y2L [m/rad]/1
  R2L/1 -> R2L [m/rad]/2
  T2L/1 -> T2L [m/m]/2
  TST_R_Disp [rad]/1 -> R2L [m/rad]/1
  TST_T_Disp [m]/1 -> T2L [m/m]/1
  Sum1/1 -> TestMass_L_Displacement [m]/1
  TST_L_Disp [m]/1 -> Sum1/1
  T2L [m/m]/1 -> Sum1/2
  EarthCurvature V2L [m/m]/1 -> Sum1/3
  R2L [m/rad]/1 -> Sum1/4
  BeamMisalignment P2L [m/rad]/1 -> Sum1/5
  BeamMisalignment Y2L [m/rad]/1 -> Sum1/6

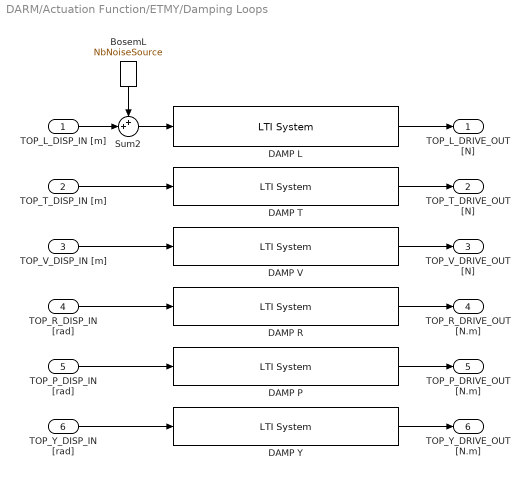
== system DARM/Actuation Function/ETMY/Damping Loops ==
  TOP_L_DISP_IN [m] : Inport
  TOP_T_DISP_IN [m] : Inport  Port=2
  TOP_V_DISP_IN [m] : Inport  Port=3
  TOP_R_DISP_IN [rad] : Inport  Port=4
  TOP_P_DISP_IN [rad] : Inport  Port=5
  TOP_Y_DISP_IN [rad] : Inport  Port=6
  BosemL : NbLibrary/NbNoiseSource  Tag=NbNoiseSource  SystemSampleTime=-1  group='BOSEM L'  asd=ifoParams.darmNb.bosem
      settings: AttributesFormatString=%<Tag>
  DAMP L : cstblocks/LTI System  SystemSampleTime=-1  sys=ifoParams.act.damp(1).ss  IC=[]
  DAMP P : cstblocks/LTI System  SystemSampleTime=-1  sys=ifoParams.act.damp(5).ss  IC=[]
  DAMP R : cstblocks/LTI System  SystemSampleTime=-1  sys=ifoParams.act.damp(4).ss  IC=[]
  DAMP T : cstblocks/LTI System  SystemSampleTime=-1  sys=ifoParams.act.damp(2).ss  IC=[]
  DAMP V : cstblocks/LTI System  SystemSampleTime=-1  sys=ifoParams.act.damp(3).ss  IC=[]
  DAMP Y : cstblocks/LTI System  SystemSampleTime=-1  sys=ifoParams.act.damp(6).ss  IC=[]
  Sum2 : Sum  Inputs=++|
  TOP_L_DRIVE_OUT [N] : Outport
  TOP_T_DRIVE_OUT [N] : Outport  Port=2
  TOP_V_DRIVE_OUT [N] : Outport  Port=3
  TOP_R_DRIVE_OUT [N.m] : Outport  Port=4
  TOP_P_DRIVE_OUT [N.m] : Outport  Port=5
  TOP_Y_DRIVE_OUT [N.m] : Outport  Port=6
  wires:
  DAMP L/1 -> TOP_L_DRIVE_OUT [N]/1
  DAMP T/1 -> TOP_T_DRIVE_OUT [N]/1
  DAMP V/1 -> TOP_V_DRIVE_OUT [N]/1
  DAMP R/1 -> TOP_R_DRIVE_OUT [N.m]/1
  DAMP P/1 -> TOP_P_DRIVE_OUT [N.m]/1
  DAMP Y/1 -> TOP_Y_DRIVE_OUT [N.m]/1
  TOP_T_DISP_IN [m]/1 -> DAMP T/1
  TOP_V_DISP_IN [m]/1 -> DAMP V/1
  TOP_R_DISP_IN [rad]/1 -> DAMP R/1
  TOP_P_DISP_IN [rad]/1 -> DAMP P/1
  TOP_Y_DISP_IN [rad]/1 -> DAMP Y/1
  BosemL/1 -> Sum2/1
  TOP_L_DISP_IN [m]/1 -> Sum2/2
  Sum2/1 -> DAMP L/1

== system DARM/Actuation Function/ETMY/Hierarchy Loops ==
  LSC_ETMY_IN [m] : Inport
  Actuator-to-Euler Transform : Subsystem
  Anti-Aliasing Chassis : Subsystem
  COILOUTF : Subsystem
  DAC : Subsystem
  Driver Electronics : Subsystem
  Driver Force Coefficient : Subsystem
  EUL2OSEM : Subsystem
  L1 LOCK : Subsystem
  L2 LOCK : Subsystem
  L3 LOCK : Subsystem
  LSC_ETMY : Subsystem
  M0 LOCK : Subsystem
  esdBias_ct : Constant  Value=ifoParams.act.esdBias_ct
  TOP_L_DRIVE_OUT [N] : Outport
  UIM_L_DRIVE_OUT [N] : Outport  Port=2
  PUM_L_DRIVE_OUT [N] : Outport  Port=3
  TST_L_DRIVE_OUT [N] : Outport  Port=4
  wires:
  Driver Force Coefficient/1(TOP_Out [N]) -> Actuator-to-Euler Transform/1(TOP_OSEM_IN [N])
  Driver Force Coefficient/2(UIM_Out [N]) -> Actuator-to-Euler Transform/2(UIM_OSEM_IN [N])
  Driver Force Coefficient/3(PUM_Out [N]) -> Actuator-to-Euler Transform/3(PUM_OSEM_IN [N])
  Driver Force Coefficient/4(TST_Out [N]) -> Actuator-to-Euler Transform/4(TST_OSEM_IN [N])
  DAC/1(TOP Out [V]) -> Anti-Aliasing Chassis/1(TOP In [V[)
  DAC/2(UIM Out [V]) -> Anti-Aliasing Chassis/2(UIM In [V])
  DAC/3(PUM Out[V]) -> Anti-Aliasing Chassis/3(PUM In [V])
  DAC/4(ESD Ctrl Out V]) -> Anti-Aliasing Chassis/4(ESD Ctrl In [V])
  DAC/5(ESD Bias Out [V]) -> Anti-Aliasing Chassis/5(ESD Bias In [V])
  COILOUTF/1(M0_OUT [ct]) -> DAC/1(M0 In [cts])
  COILOUTF/2(L1_OUT [ct]) -> DAC/2(L1 In [cts])
  COILOUTF/3(L2_OUT [ct]) -> DAC/3(L2 In [cts])
  COILOUTF/4(L3_CTRL_OUT [ct]) -> DAC/4(L3 Ctrl In [cts])
  COILOUTF/5(L3_BIAS_OUT [ct]) -> DAC/5(L3 Bias In [cts])
  M0 LOCK/1(M0_OUT [ct]) -> EUL2OSEM/1(M0_L_IN [ct])
  EUL2OSEM/1(M0_OSEM_OUT [ct]) -> COILOUTF/1(M0_IN [ct])
  EUL2OSEM/2(L1_OSEM_OUT [ct]) -> COILOUTF/2(L1_IN [ct])
  EUL2OSEM/3(L2_OSEM_OUT [ct]) -> COILOUTF/3(L2_IN [ct])
  EUL2OSEM/4(L3_OSEM_OUT [ct]) -> COILOUTF/4(L3_CTRL_IN [ct])
  esdBias_ct/1 -> COILOUTF/5(L3_BIAS_IN [ct])
  LSC_ETMY_IN [m]/1 -> LSC_ETMY/1(LSC_ETMX_IN)
  Actuator-to-Euler Transform/1(TOP_L_OUT [N]) -> TOP_L_DRIVE_OUT [N]/1
  Actuator-to-Euler Transform/2(UIM_L_OUT [N]) -> UIM_L_DRIVE_OUT [N]/1
  Actuator-to-Euler Transform/3(PUM_L_OUT [N]) -> PUM_L_DRIVE_OUT [N]/1
  Actuator-to-Euler Transform/4(TST_L_OUT [N]) -> TST_L_DRIVE_OUT [N]/1
  Anti-Aliasing Chassis/1(TOP Out [V]) -> Driver Electronics/1(TOP In [V])
  Anti-Aliasing Chassis/2(UIM Out [V]) -> Driver Electronics/2(UIM In [V])
  Anti-Aliasing Chassis/3(PUM Out[V]) -> Driver Electronics/3(PUM In [V])
  Anti-Aliasing Chassis/4(ESD Ctrl Out V]) -> Driver Electronics/4(ESD Ctrl In [V])
  Anti-Aliasing Chassis/5(ESD Bias Out [V]) -> Driver Electronics/5(ESD Bias In [V])
  Driver Electronics/1(TOP Out [A]) -> Driver Force Coefficient/1(In1[A])
  Driver Electronics/2(UIM Out [A]) -> Driver Force Coefficient/2(In2[A])
  Driver Electronics/3(PUM Out [A]) -> Driver Force Coefficient/3(In3[A])
  Driver Electronics/4(ESD Ctrl Out[V]) -> Driver Force Coefficient/4(Vsig[V])
  Driver Electronics/5(ESD Bias Out[V]) -> Driver Force Coefficient/5(Vbias[V])
  L1 LOCK/1(L1_OUT [ct]) -> EUL2OSEM/2(L1_L_IN [ct])
  L2 LOCK/1(L2_OUT [ct]) -> EUL2OSEM/3(L2_L_IN [ct])
  L3 LOCK/1(L3_OUT [ct]) -> EUL2OSEM/4(L3_L_IN [ct])
  LSC_ETMY/1("LSC_ETMX_OUT ") -> M0 LOCK/1(LSC_IN [m]), L1 LOCK/1(LSC_IN [m]), L2 LOCK/1(LSC_IN [m]), L3 LOCK/1(LSC_IN [m])

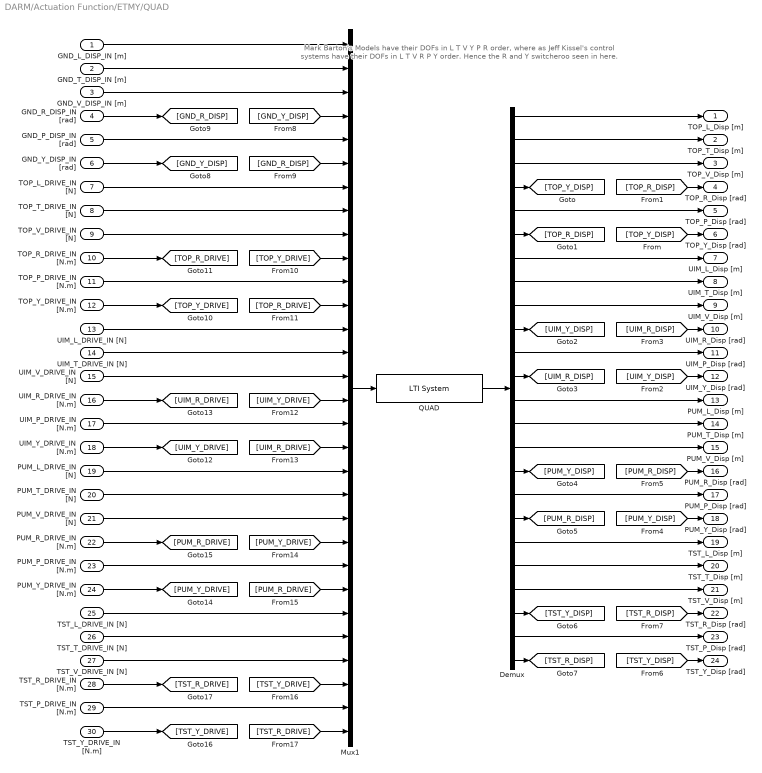
== system DARM/Actuation Function/ETMY/QUAD ==
  note: Mark Barton's Models have their DOFs in
      | L T V Y P R order, where as Jeff Kissel's control
      | systems have their DOFs in  L T V R P Y order.
      | Hence the R and Y switcheroo seen in here.
  GND_L_DISP_IN [m] : Inport
  GND_T_DISP_IN [m] : Inport  Port=2
  GND_V_DISP_IN [m] : Inport  Port=3
  GND_R_DISP_IN [rad] : Inport  Port=4
  GND_P_DISP_IN [rad] : Inport  Port=5
  GND_Y_DISP_IN [rad] : Inport  Port=6
  TOP_L_DRIVE_IN [N] : Inport  Port=7
  TOP_T_DRIVE_IN [N] : Inport  Port=8
  TOP_V_DRIVE_IN [N] : Inport  Port=9
  TOP_R_DRIVE_IN [N.m] : Inport  Port=10
  TOP_P_DRIVE_IN [N.m] : Inport  Port=11
  TOP_Y_DRIVE_IN [N.m] : Inport  Port=12
  UIM_L_DRIVE_IN [N] : Inport  Port=13
  UIM_T_DRIVE_IN [N] : Inport  Port=14
  UIM_V_DRIVE_IN [N] : Inport  Port=15
  UIM_R_DRIVE_IN [N.m] : Inport  Port=16
  UIM_P_DRIVE_IN [N.m] : Inport  Port=17
  UIM_Y_DRIVE_IN [N.m] : Inport  Port=18
  PUM_L_DRIVE_IN [N] : Inport  Port=19
  PUM_T_DRIVE_IN [N] : Inport  Port=20
  PUM_V_DRIVE_IN [N] : Inport  Port=21
  PUM_R_DRIVE_IN [N.m] : Inport  Port=22
  PUM_P_DRIVE_IN [N.m] : Inport  Port=23
  PUM_Y_DRIVE_IN [N.m] : Inport  Port=24
  TST_L_DRIVE_IN [N] : Inport  Port=25
  TST_T_DRIVE_IN [N] : Inport  Port=26
  TST_V_DRIVE_IN [N] : Inport  Port=27
  TST_R_DRIVE_IN [N.m] : Inport  Port=28
  TST_P_DRIVE_IN [N.m] : Inport  Port=29
  TST_Y_DRIVE_IN [N.m] : Inport  Port=30
  Demux : Demux  Outputs=24
  Mux1 : Mux  Inputs=30
  QUAD : cstblocks/LTI System  Description=FlexTf: ifoParams.act.quadModel.frd  SystemSampleTime=-1  sys=ifoParams.act.quadModel.ss  IC=[]
      settings: AttributesFormatString=%<Description>
  TOP_L_Disp [m] : Outport
  TOP_T_Disp [m] : Outport  Port=2
  TOP_V_Disp [m] : Outport  Port=3
  TOP_R_Disp [rad] : Outport  Port=4
  TOP_P_Disp [rad] : Outport  Port=5
  TOP_Y_Disp [rad] : Outport  Port=6
  UIM_L_Disp [m] : Outport  Port=7
  UIM_T_Disp [m] : Outport  Port=8
  UIM_V_Disp [m] : Outport  Port=9
  UIM_R_Disp [rad] : Outport  Port=10
  UIM_P_Disp [rad] : Outport  Port=11
  UIM_Y_Disp [rad] : Outport  Port=12
  PUM_L_Disp [m] : Outport  Port=13
  PUM_T_Disp [m] : Outport  Port=14
  PUM_V_Disp [m] : Outport  Port=15
  PUM_R_Disp [rad] : Outport  Port=16
  PUM_P_Disp [rad] : Outport  Port=17
  PUM_Y_Disp [rad] : Outport  Port=18
  TST_L_Disp [m] : Outport  Port=19
  TST_T_Disp [m] : Outport  Port=20
  TST_V_Disp [m] : Outport  Port=21
  TST_R_Disp [rad] : Outport  Port=22
  TST_P_Disp [rad] : Outport  Port=23
  TST_Y_Disp [rad] : Outport  Port=24
  wires:
  QUAD/1 -> Demux/1
  Mux1/1 -> QUAD/1
  GND_L_DISP_IN [m]/1 -> Mux1/1
  GND_T_DISP_IN [m]/1 -> Mux1/2
  GND_V_DISP_IN [m]/1 -> Mux1/3
  Demux/1 -> TOP_L_Disp [m]/1
  Demux/2 -> TOP_T_Disp [m]/1
  Demux/3 -> TOP_V_Disp [m]/1
  TOP_L_DRIVE_IN [N]/1 -> Mux1/7
  TOP_T_DRIVE_IN [N]/1 -> Mux1/8
  TOP_V_DRIVE_IN [N]/1 -> Mux1/9
  Demux/7 -> UIM_L_Disp [m]/1
  Demux/8 -> UIM_T_Disp [m]/1
  Demux/9 -> UIM_V_Disp [m]/1
  UIM_T_DRIVE_IN [N]/1 -> Mux1/14
  UIM_V_DRIVE_IN [N]/1 -> Mux1/15
  Demux/13 -> PUM_L_Disp [m]/1
  Demux/14 -> PUM_T_Disp [m]/1
  Demux/15 -> PUM_V_Disp [m]/1
  PUM_L_DRIVE_IN [N]/1 -> Mux1/19
  PUM_T_DRIVE_IN [N]/1 -> Mux1/20
  PUM_V_DRIVE_IN [N]/1 -> Mux1/21
  Demux/19 -> TST_L_Disp [m]/1
  Demux/20 -> TST_T_Disp [m]/1
  Demux/21 -> TST_V_Disp [m]/1
  TST_L_DRIVE_IN [N]/1 -> Mux1/25
  TST_T_DRIVE_IN [N]/1 -> Mux1/26
  TST_V_DRIVE_IN [N]/1 -> Mux1/27
  Demux/4 -> [TOP_Y_DISP]
  [TOP_Y_DISP] -> TOP_Y_Disp [rad]/1
  Demux/6 -> [TOP_R_DISP]
  [TOP_R_DISP] -> TOP_R_Disp [rad]/1
  Demux/5 -> TOP_P_Disp [rad]/1
  Demux/10 -> [UIM_Y_DISP]
  Demux/11 -> UIM_P_Disp [rad]/1
  [UIM_R_DISP] -> UIM_R_Disp [rad]/1
  Demux/12 -> [UIM_R_DISP]
  [UIM_Y_DISP] -> UIM_Y_Disp [rad]/1
  Demux/16 -> [PUM_Y_DISP]
  [PUM_R_DISP] -> PUM_R_Disp [rad]/1
  Demux/17 -> PUM_P_Disp [rad]/1
  Demux/18 -> [PUM_R_DISP]
  [PUM_Y_DISP] -> PUM_Y_Disp [rad]/1
  [TST_R_DISP] -> TST_R_Disp [rad]/1
  Demux/22 -> [TST_Y_DISP]
  Demux/23 -> TST_P_Disp [rad]/1
  Demux/24 -> [TST_R_DISP]
  [TST_Y_DISP] -> TST_Y_Disp [rad]/1
  UIM_L_DRIVE_IN [N]/1 -> Mux1/13
  GND_R_DISP_IN [rad]/1 -> [GND_R_DISP]
  [GND_Y_DISP] -> Mux1/4
  GND_P_DISP_IN [rad]/1 -> Mux1/5
  GND_Y_DISP_IN [rad]/1 -> [GND_Y_DISP]
  [GND_R_DISP] -> Mux1/6
  TOP_R_DRIVE_IN [N.m]/1 -> [TOP_R_DRIVE]
  TOP_P_DRIVE_IN [N.m]/1 -> Mux1/11
  TOP_Y_DRIVE_IN [N.m]/1 -> [TOP_Y_DRIVE]
  [TOP_Y_DRIVE] -> Mux1/10
  [TOP_R_DRIVE] -> Mux1/12
  UIM_R_DRIVE_IN [N.m]/1 -> [UIM_R_DRIVE]
  UIM_Y_DRIVE_IN [N.m]/1 -> [UIM_Y_DRIVE]
  PUM_R_DRIVE_IN [N.m]/1 -> [PUM_R_DRIVE]
  PUM_Y_DRIVE_IN [N.m]/1 -> [PUM_Y_DRIVE]
  TST_R_DRIVE_IN [N.m]/1 -> [TST_R_DRIVE]
  TST_Y_DRIVE_IN [N.m]/1 -> [TST_Y_DRIVE]
  [UIM_Y_DRIVE] -> Mux1/16
  UIM_P_DRIVE_IN [N.m]/1 -> Mux1/17
  [UIM_R_DRIVE] -> Mux1/18
  [PUM_Y_DRIVE] -> Mux1/22
  PUM_P_DRIVE_IN [N.m]/1 -> Mux1/23
  [PUM_R_DRIVE] -> Mux1/24
  [TST_Y_DRIVE] -> Mux1/28
  TST_P_DRIVE_IN [N.m]/1 -> Mux1/29
  [TST_R_DRIVE] -> Mux1/30

== system DARM/Sensing Function/DCPD Analog Electronics/Anti-Aliasing Chassis ==
  PD1_IN1 [V] : Inport
  PD2_IN [V] : Inport  Port=2
  Gain1 : Gain
  Gain3 : Gain
  PD1_OUT [V] : Outport
  PD2_OUT [V] : Outport  Port=2
  wires:
  PD1_IN1 [V]/1 -> Gain3/1
  Gain3/1 -> PD1_OUT [V]/1
  PD2_IN [V]/1 -> Gain1/1
  Gain1/1 -> PD2_OUT [V]/1

== system DARM/Sensing Function/DCPD Analog Electronics/PD Quantum Efficiency ==
  PD1_IN1 [W] : Inport
  PD2_IN [W] : Inport  Port=2
  Gain1 : Gain  Gain=ifoParams.sens.pdQuantumEfficiency
  Gain3 : Gain  Gain=ifoParams.sens.pdQuantumEfficiency
  PD1_OUT [A] : Outport
  PD2_OUT [A] : Outport  Port=2
  wires:
  PD1_IN1 [W]/1 -> Gain3/1
  Gain3/1 -> PD1_OUT [A]/1
  PD2_IN [W]/1 -> Gain1/1
  Gain1/1 -> PD2_OUT [A]/1

== system DARM/Sensing Function/DCPD Analog Electronics/Preamps ==
  PD1_IN1 [A] : Inport
  PD2_IN [A] : Inport  Port=2
  Preamp_PD1 : Subsystem
  Preamp_PD2 : Subsystem
  PD1_OUT [V] : Outport
  PD2_OUT [V] : Outport  Port=2
  wires:
  PD1_IN1 [A]/1 -> Preamp_PD1/1(In [A])
  Preamp_PD1/1(Out [V]) -> PD1_OUT [V]/1
  PD2_IN [A]/1 -> Preamp_PD2/1(In [A])
  Preamp_PD2/1(Out [V]) -> PD2_OUT [V]/1

== system DARM/Sensing Function/DCPD Analog Electronics/Whitening Chassis ==
  PD1_IN1 [V] : Inport
  PD2_IN [V] : Inport  Port=2
  Whitening_PD1 : Subsystem
  Whitening_PD2 : Subsystem
  PD1_OUT [V] : Outport
  PD2_OUT [V] : Outport  Port=2
  wires:
  PD1_IN1 [V]/1 -> Whitening_PD1/1(In [V])
  Whitening_PD1/1(Out [V]) -> PD1_OUT [V]/1
  PD2_IN [V]/1 -> Whitening_PD2/1(In [V])
  Whitening_PD2/1(Out [V]) -> PD2_OUT [V]/1

== system DARM/Sensing Function/DCPD Signal Conditioning/64k to 16k Downsampling Filter ==
  PDq_IN [ct] : Inport
  PD2_IN [ct] : Inport  Port=2
  cdsDownSamplingFilter_64kto16k_PD1 : cstblocks/LTI System  SystemSampleTime=-1  sys=ifoParams.sens.cdsDownsamplingFilter_64kto16k.ss  IC=[]
  cdsDownSamplingFilter_64kto16k_PD2 : cstblocks/LTI System  SystemSampleTime=-1  sys=ifoParams.sens.cdsDownsamplingFilter_64kto16k.ss  IC=[]
  PD1_OUT [ct] : Outport
  PD2_OUT [ct] : Outport  Port=2
  wires:
  PDq_IN [ct]/1 -> cdsDownSamplingFilter_64kto16k_PD1/1
  cdsDownSamplingFilter_64kto16k_PD1/1 -> PD1_OUT [ct]/1
  PD2_IN [ct]/1 -> cdsDownSamplingFilter_64kto16k_PD2/1
  cdsDownSamplingFilter_64kto16k_PD2/1 -> PD2_OUT [ct]/1

== system DARM/Sensing Function/DCPD Signal Conditioning/ISCINF ==
  PD1_IN [ct] : Inport
  PD2_IN [ct] : Inport  Port=2
  AntiPreamps_PD1 : Subsystem
  AntiPreamps_PD2 : Subsystem
  AntiWhitening_PD1 : Subsystem
  AntiWhitening_PD2 : Subsystem
  PD1_OUT [m] : Outport
  PD2_OUT [m] : Outport  Port=2
  wires:
  PD1_IN [ct]/1 -> AntiPreamps_PD1/1(In [ct])
  AntiWhitening_PD1/1(Out [ct]) -> PD1_OUT [m]/1
  PD2_IN [ct]/1 -> AntiPreamps_PD2/1(In [ct])
  AntiWhitening_PD2/1(Out [ct]) -> PD2_OUT [m]/1
  AntiPreamps_PD1/1(Out [ct]) -> AntiWhitening_PD1/1(In [ct])
  AntiPreamps_PD2/1(Out [ct]) -> AntiWhitening_PD2/1(In [ct])

== system DARM/Actuation Function/ETMX/Hierarchy Loops/Actuator-to-Euler Transform ==
  note: 4 coil-magnet
      | actuators
  note: 4 coil-magnet
      | actuators
  note: 2 coil-magnet
      | actuators
  note: 4 ESD Quadrants
  TOP_OSEM_IN [N] : Inport
  UIM_OSEM_IN [N] : Inport  Port=2
  PUM_OSEM_IN [N] : Inport  Port=3
  TST_OSEM_IN [N] : Inport  Port=4
  Gain1 : Gain  Gain=4
  Gain3 : Gain  Gain=2
  Gain4 : Gain  Gain=4
  Gain5 : Gain  Gain=4
  TOP_L_OUT [N] : Outport
  UIM_L_OUT [N] : Outport  Port=2
  PUM_L_OUT [N] : Outport  Port=3
  TST_L_OUT [N] : Outport  Port=4
  wires:
  TOP_OSEM_IN [N]/1 -> Gain3/1
  Gain3/1 -> TOP_L_OUT [N]/1
  UIM_OSEM_IN [N]/1 -> Gain4/1
  Gain4/1 -> UIM_L_OUT [N]/1
  PUM_OSEM_IN [N]/1 -> Gain5/1
  Gain5/1 -> PUM_L_OUT [N]/1
  TST_OSEM_IN [N]/1 -> Gain1/1
  Gain1/1 -> TST_L_OUT [N]/1

== system DARM/Actuation Function/ETMX/Hierarchy Loops/Anti-Aliasing Chassis ==
  TOP In [V[ : Inport
  UIM In [V] : Inport  Port=2
  PUM In [V] : Inport  Port=3
  ESD Ctrl In [V] : Inport  Port=4
  ESD Bias In [V] : Inport  Port=5
  Gain{,1..4} (5 alike) : Gain
  TOP Out [V] : Outport
  UIM Out [V] : Outport  Port=2
  PUM Out[V] : Outport  Port=3
  ESD Ctrl Out V] : Outport  Port=4
  ESD Bias Out [V] : Outport  Port=5
  wires:
  Gain1/1 -> UIM Out [V]/1
  UIM In [V]/1 -> Gain1/1
  Gain2/1 -> PUM Out[V]/1
  PUM In [V]/1 -> Gain2/1
  Gain/1 -> TOP Out [V]/1
  TOP In [V[/1 -> Gain/1
  Gain3/1 -> ESD Ctrl Out V]/1
  ESD Ctrl In [V]/1 -> Gain3/1
  Gain4/1 -> ESD Bias Out [V]/1
  ESD Bias In [V]/1 -> Gain4/1

== system DARM/Actuation Function/ETMX/Hierarchy Loops/COILOUTF ==
  note: See T1100378 and LLO aLOG 4495 for reference
  M0_IN [ct] : Inport
  L1_IN [ct] : Inport  Port=2
  L2_IN [ct] : Inport  Port=3
  L3_CTRL_IN [ct] : Inport  Port=4
  L3_BIAS_IN [ct] : Inport  Port=5
  L1 : Subsystem
  L2 : Subsystem
  L3 : Subsystem
  M0 : Subsystem
  M0_OUT [ct] : Outport
  L1_OUT [ct] : Outport  Port=2
  L2_OUT [ct] : Outport  Port=3
  L3_CTRL_OUT [ct] : Outport  Port=4
  L3_BIAS_OUT [ct] : Outport  Port=5
  wires:
  M0/1(Out [ct]) -> M0_OUT [ct]/1
  M0_IN [ct]/1 -> M0/1(In [ct])
  L2_IN [ct]/1 -> L2/1(In [ct])
  L1_IN [ct]/1 -> L1/1(In [ct])
  L3/1(Ctrl Out [V]) -> L3_CTRL_OUT [ct]/1
  L3_CTRL_IN [ct]/1 -> L3/1(Ctrl In [V])
  L1/1(Out [ct]) -> L1_OUT [ct]/1
  L2/1(Out [ct]) -> L2_OUT [ct]/1
  L3/2(Bias Out [V]) -> L3_BIAS_OUT [ct]/1
  L3_BIAS_IN [ct]/1 -> L3/2(Bias In [V])

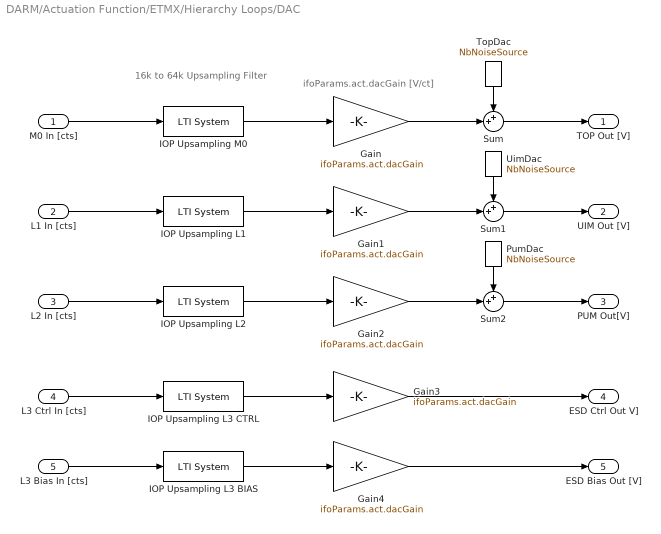
== system DARM/Actuation Function/ETMX/Hierarchy Loops/DAC ==
  note: ifoParams.act.dacGain
      | [V/ct]
  note: 16k to 64k Upsampling Filter
  M0 In [cts] : Inport
  L1 In [cts] : Inport  Port=2
  L2 In [cts] : Inport  Port=3
  L3 Ctrl In [cts] : Inport  Port=4
  L3 Bias In [cts] : Inport  Port=5
  Gain{,1..4} (5 alike) : Gain  Gain=ifoParams.act.dacGain
  IOP Upsampling L1 : cstblocks/LTI System  SystemSampleTime=-1  sys=ifoParams.act.cdsUpsamplingFilter_16kto64k.ss  IC=[]
  IOP Upsampling L2 : cstblocks/LTI System  SystemSampleTime=-1  sys=ifoParams.act.cdsUpsamplingFilter_16kto64k.ss  IC=[]
  IOP Upsampling L3 BIAS : cstblocks/LTI System  SystemSampleTime=-1  sys=ifoParams.act.cdsUpsamplingFilter_16kto64k.ss  IC=[]
  IOP Upsampling L3 CTRL : cstblocks/LTI System  SystemSampleTime=-1  sys=ifoParams.act.cdsUpsamplingFilter_16kto64k.ss  IC=[]
  IOP Upsampling M0 : cstblocks/LTI System  SystemSampleTime=-1  sys=ifoParams.act.cdsUpsamplingFilter_16kto64k.ss  IC=[]
  PumDac : NbLibrary/NbNoiseSource  Tag=NbNoiseSource  SystemSampleTime=-1  group='QUAD Actuator'  asd=ifoParams.darmNb.quadPumDac
      settings: AttributesFormatString=%<Tag>
  Sum : Sum  Inputs=++|
  Sum1 : Sum  Inputs=++|
  Sum2 : Sum  Inputs=++|
  TopDac : NbLibrary/NbNoiseSource  Tag=NbNoiseSource  SystemSampleTime=-1  group='QUAD Actuator'  asd=ifoParams.darmNb.quadTopDac
      settings: AttributesFormatString=%<Tag>
  UimDac : NbLibrary/NbNoiseSource  Tag=NbNoiseSource  SystemSampleTime=-1  group='QUAD Actuator'  asd=ifoParams.darmNb.quadUimDac
      settings: AttributesFormatString=%<Tag>
  TOP Out [V] : Outport
  UIM Out [V] : Outport  Port=2
  PUM Out[V] : Outport  Port=3
  ESD Ctrl Out V] : Outport  Port=4
  ESD Bias Out [V] : Outport  Port=5
  wires:
  L1 In [cts]/1 -> IOP Upsampling L1/1
  L2 In [cts]/1 -> IOP Upsampling L2/1
  L3 Ctrl In [cts]/1 -> IOP Upsampling L3 CTRL/1
  Gain4/1 -> ESD Bias Out [V]/1
  L3 Bias In [cts]/1 -> IOP Upsampling L3 BIAS/1
  M0 In [cts]/1 -> IOP Upsampling M0/1
  IOP Upsampling M0/1 -> Gain/1
  IOP Upsampling L1/1 -> Gain1/1
  IOP Upsampling L2/1 -> Gain2/1
  IOP Upsampling L3 CTRL/1 -> Gain3/1
  IOP Upsampling L3 BIAS/1 -> Gain4/1
  Gain/1 -> Sum/2
  Sum/1 -> TOP Out [V]/1
  TopDac/1 -> Sum/1
  Gain1/1 -> Sum1/2
  UimDac/1 -> Sum1/1
  Sum1/1 -> UIM Out [V]/1
  Gain2/1 -> Sum2/2
  PumDac/1 -> Sum2/1
  Sum2/1 -> PUM Out[V]/1
  Gain3/1 -> ESD Ctrl Out V]/1
